simulink model "Pouziti_Maticove_vs_poprvcich"  (R2020b)
settings: Solver=VariableStepAuto  StartTime=0.0  StopTime=10.0  RelTol=1e-3  EnableMultiTasking=on
settings Model: Creator=Jirkovsk  LastModifiedBy=jirkovsky
settings DataIOCC: LimitDataPoints=on  SaveFormat=Array  SignalLoggingSaveFormat=ModelDataLogs  ReturnWorkspaceOutputs=off
settings OptimizationCC: ExpressionDepthLimit=2147483647  InitFltsAndDblsToZero=on  LifeSpan=inf
settings DebuggingCC: UnderspecifiedInitializationDetection=Classic  MergeDetectMultiDrivingBlocksExec=none  SolverPrmCheckMsg=warning  FcnCallInpInsideContextMsg=warning  StateNameClashWarn=warning  SFUnexpectedBacktrackingDiag=warning  SFNoUnconditionalDefaultTransitionDiag=warning  SFExecutionAtInitializationDiag=none  ArithmeticOperatorsInVariantConditions=warning
settings HardwareCC: ProdBitPerPointer=32  ProdBitPerSizeT=32  ProdBitPerPtrDiffT=32  ProdLargestAtomicFloat=None  ProdIntDivRoundTo=Undefined  ProdEndianess=Unspecified  ProdWordSize=32  ProdHWDeviceType=32-bit Generic
settings ModelReferenceCC: PropagateSignalLabelsOutOfModel=off
settings SFSimCC: SimUseLocalCustomCode=off  CustomCodeUndefinedFunction=UseInterfaceOnly
settings RTWCC: RTWUseLocalCustomCode=off
settings CodeAppCC: StateflowObjectComments=on
settings GRTTargetCC: TargetLangStandard=C89/C90 (ANSI)  CombineOutputUpdateFcns=off  GRTInterface=on
settings ConfigComp: CovMetricSettings=dw  CovSaveCumulativeToWorkspaceVar=on  CovSaveSingleToWorkspaceVar=on  CovExternalEMLEnable=off  CovSFcnEnable=off

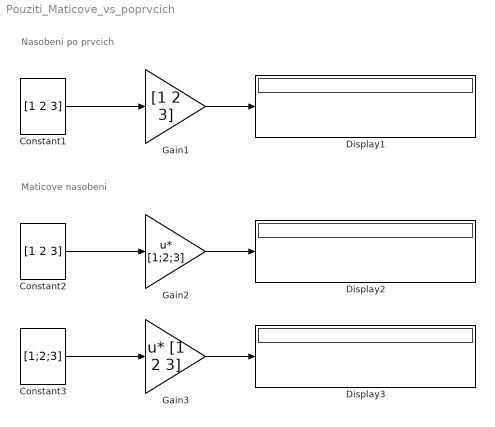
== system Pouziti_Maticove_vs_poprvcich ==
  note: Nasobeni po prvcich
  note: Maticove nasobeni
  Constant1 : Constant  Value=[1 2 3]  VectorParams1D=off
  Constant2 : Constant  Value=[1 2 3]  VectorParams1D=off
  Constant3 : Constant  Value=[1;2;3]  VectorParams1D=off
  Display1 : Display
  Display2 : Display
  Display3 : Display
  Gain1 : Gain  Gain=[1 2 3]
  Gain2 : Gain  Gain=[1;2;3]  Multiplication=Matrix(u*K)
  Gain3 : Gain  Gain=[1 2 3]  Multiplication=Matrix(u*K)
  wires:
  Gain1/1 -> Display1/1
  Constant1/1 -> Gain1/1
  Gain2/1 -> Display2/1
  Constant2/1 -> Gain2/1
  Gain3/1 -> Display3/1
  Constant3/1 -> Gain3/1
